simulink model "pH_Neut"  (Simulink 7.8)
settings: Solver=FixedStepDiscrete  StartTime=0.0  StopTime=1  FixedStep=0.005  RelTol=1e-5  AbsTol=1e-5
undefined symbols (not defined in the file): up
settings Model: Creator=pmahapatra  LastModifiedBy=pmahapatra
settings OptimizationCC: BlockReduction=off  BooleanDataType=off  InlineInvariantSignals=on  InitFltsAndDblsToZero=on
settings DebuggingCC: SaveWithParameterizedLinksMsg=none  SignalResolutionControl=TryResolveAllWithWarning  SolverPrmCheckMsg=none  MultiTaskDSMMsg=warning  MultiTaskCondExecSysMsg=none  FcnCallInpInsideContextMsg=Use local settings  StrictBusMsg=None
settings RTWCC: IncludeERTFirstTime=on
settings GRTTargetCC: TargetFcnLib=ansi_tfl_tmw.mat

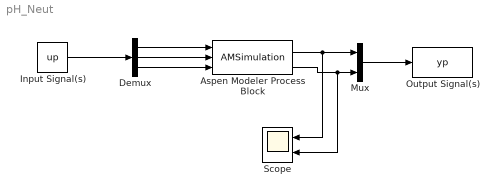
== system pH_Neut ==
  Aspen Modeler Process Block : M-S-Function  LoadFcn=|  FunctionName=AMSimulation  Parameters='E:\PROJECTS\CCSI\Dynamic ROMS\ACM_PH\pH_Neut.acmf','ACM Application',3,'B1.Feed1.F|m3/hr\B1.Feed2.F|m3/hr\B1.Feed3.F|m3/hr',2,'B1.PH\B1.Prod.Ca|kmol/m3',true,false,true
      | LoadModel=actxserver('AMSimulation.Control');
      | invoke(LoadModel,'LoadModel',get_param(gcb,'Parameters'),pwd);
      | LoadModel.delete;
      settings: DeleteFcn=|
      | CloseModel=actxserver('AMSimulation.Control');
      | invoke(CloseModel,'CloseModel',get_param(gcb,'Parameters'));
      | CloseModel.delete;
      settings: OpenFcn=|
      | SetupGUI=actxserver('AMSimulation.Setup');
      | NewParam=invoke(SetupGUI,'SetupModel',get_param(gcb,'Parameters'),pwd,get_param(gcb,'Name'));
      | set_param(gcb,'Parameters',NewParam);
      | SetupGUI.delete;
  Demux : Demux  Outputs=3
  Input Signal(s) : Constant  Value=up
  Mux : Mux  Inputs=2
  Output Signal(s) : ToWorkspace  VariableName=yp  SampleTime=-1  SaveFormat=Array
  Scope : Scope  NumInputPorts=2
      settings: YMin=-5~-5  YMax=5~5
  wires:
  Demux/1 -> Aspen Modeler Process Block/1
  Demux/2 -> Aspen Modeler Process Block/2
  Demux/3 -> Aspen Modeler Process Block/3
  Input Signal(s)/1 -> Demux/1
  Aspen Modeler Process Block/1 -> Mux/1, Scope/1
  Aspen Modeler Process Block/2 -> Mux/2, Scope/2
  Mux/1 -> Output Signal(s)/1
